simulink model "generator_controls"  (R2021b)
settings: Solver=VariableStepAuto  StartTime=0.0  StopTime=10.0  RelTol=1e-3
libraries: customLib x4, spsAC1AExcitationSystemLib x1, spsDC1AExcitationSystemLib x1, spsST1AExcitationSystemLib x1, eeGovernorG1 x1, eeSmPSS1A x1, eeSmPSS2C x1
settings Model: Creator=JoEn  LastModifiedBy=ah4430
settings DebuggingCC: UnconnectedInputMsg=none  UnconnectedOutputMsg=none  UnconnectedLineMsg=none
settings ModelReferenceCC: EnableRefExpFcnMdlSchedulingChecks=off
settings RTWCC: DLArmComputeVersion=20.02.1

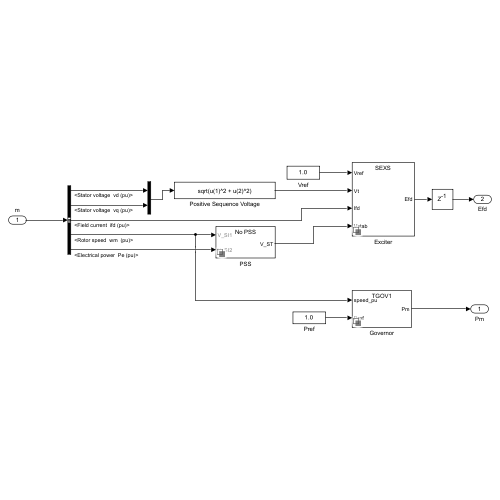
[thumbnail: Simulink's stored preview of the top-level diagram]
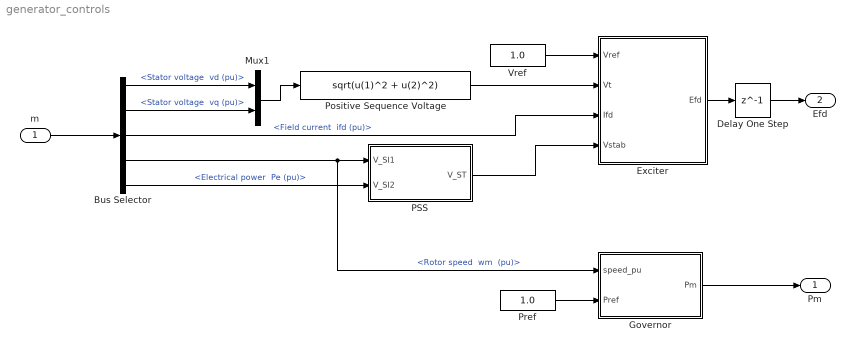
== system generator_controls ==
  m : Inport
  Bus Selector : BusSelector  OutputSignals="dq0 components.Stator voltage  vd (pu),dq0 components.Stator voltage  vq (pu),dq0 components.Field current  ifd (pu),Mechanical.Rotor speed  wm  (pu),Mechanical.Electrical power  Pe (pu)"
  Delay One Step : Delay  DelayLength=1
  Exciter : Subsystem  Variant=on  VariantControlMode=label  LabelModeActiveChoice=sexs
  Governor : Subsystem  Variant=on  VariantControlMode=label  LabelModeActiveChoice=tgov1
  Mux1 : Mux  Inputs=2
  PSS : Subsystem  Variant=on  VariantControlMode=label  LabelModeActiveChoice=none
  Positive Sequence Voltage : Fcn  Expr=sqrt(u(1)^2 + u(2)^2)
  Pref : Constant  Value=1.0
  Vref : Constant  Value=1.0
  Pm : Outport
  Efd : Outport  Port=2
  wires:
  Bus Selector/2 -> Mux1/2  "<Stator voltage  vq (pu)>"
  Vref/1 -> Exciter/1(Vref)
  Delay One Step/1 -> Efd/1
  Bus Selector/3 -> Exciter/3(Ifd)  "<Field current  ifd (pu)>"
  PSS/1(V_ST) -> Exciter/4(Vstab)
  Mux1/1 -> Positive Sequence Voltage/1
  Exciter/1(Efd) -> Delay One Step/1
  Pref/1 -> Governor/2(Pref)
  Governor/1(Pm) -> Pm/1
  Positive Sequence Voltage/1 -> Exciter/2(Vt)
  Bus Selector/1 -> Mux1/1  "<Stator voltage  vd (pu)>"
  m/1 -> Bus Selector/1
  Bus Selector/4 -> Governor/1(speed_pu), PSS/1(V_SI1)  "<Rotor speed  wm  (pu)>"
  Bus Selector/5 -> PSS/2(V_SI2)  "<Electrical power  Pe (pu)>"

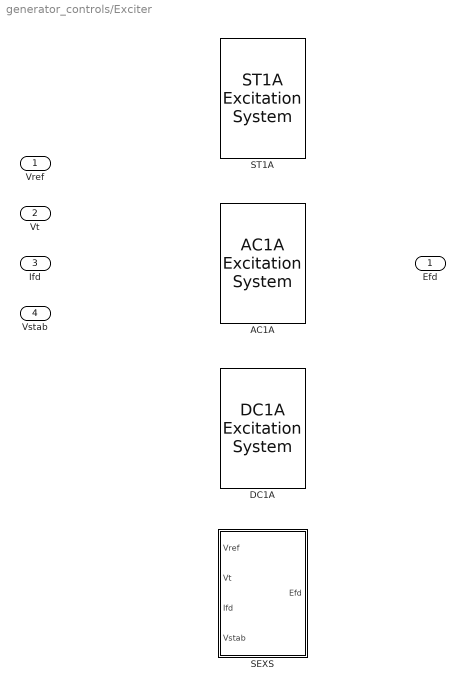
== system generator_controls/Exciter ==
  Vref : Inport
  Vt : Inport  Port=2
  Ifd : Inport  Port=3
  Vstab : Inport  Port=4
  AC1A : spsAC1AExcitationSystemLib/AC1A Excitation System  VariantControl=ac1a  Tr=20e-3  KaTa=[400 0.02]  VAminmax=[-14.5 14.5]  VRminmax=[-5.43 6.03]  KfTf=[0.03 1.0]  TbTc=[0 0]  KeTe=[1.0 0.80]  Ve12=[4.18 3.14]  SeVe12=[0.10 0.03]  Kd=0.38  Kc=0.20  v0=[1.025 1.5083]  TsBlock=0
  DC1A : spsDC1AExcitationSystemLib/DC1A Excitation System  VariantControl=dc1a  Tr=1e-6  KaTa=[20 0.2]  VRminmax=[-5 5]  KfTf=[0.063 0.35]  TbTc=[0 0]  KeTe=[1.0 0.314]  Efd12=[4.5 3.3]  SeEfd12=[4.2662 0.6602]  v0=[1.025 1.5083]  TsBlock=0
  SEXS : Subsystem  VariantControl=sexs
  ST1A : spsST1AExcitationSystemLib/ST1A Excitation System  VariantControl=st1a  Tr=20e-3  KaTa=[210 0.001]  VIminmax=[-999 +999]  VAminmax=[-999 999]  VRminmax=[-6.0 6.43]  KfTf=[0.001 1]  TbTc=[0 0 0 0]  KLR=1  ILR=2  Kc=0.038  v0=[1 1]  TsBlock=0
  Efd : Outport

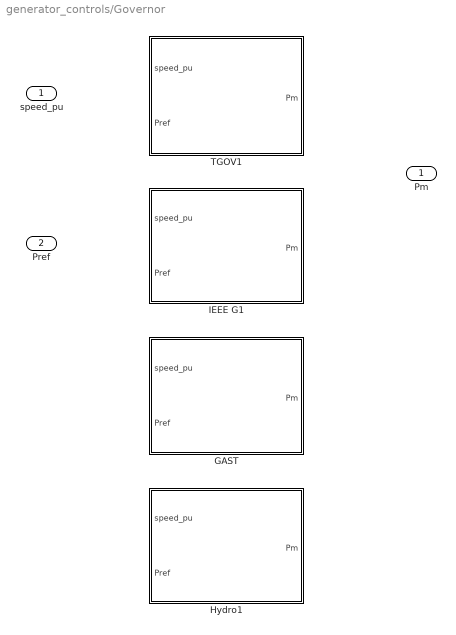
== system generator_controls/Governor ==
  speed_pu : Inport
  Pref : Inport  Port=2
  GAST : Subsystem  VariantControl=gast
  Hydro1 : Subsystem  VariantControl=hydro1
  IEEE G1 : Subsystem  VariantControl=ieeeg1
  TGOV1 : Subsystem  VariantControl=tgov1
  Pm : Outport

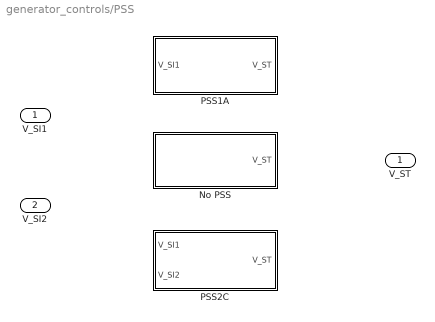
== system generator_controls/PSS ==
  V_SI1 : Inport
  V_SI2 : Inport  Port=2
  No PSS : Subsystem  VariantControl=none
  PSS1A : Subsystem  VariantControl=pss1a
  PSS2C : Subsystem  VariantControl=pss2c
  V_ST : Outport

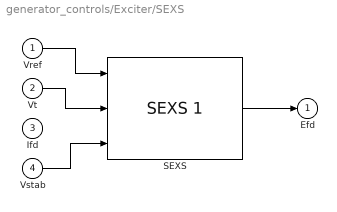
== system generator_controls/Exciter/SEXS ==
  Vref : Inport
  Vt : Inport  Port=2
  Ifd : Inport  Port=3
  Vstab : Inport  Port=4
  SEXS : customLib/SEXS 1  TA=0  TB=0  K=0  TE=0  Emin=0  Emax=0
      settings: SourceProductName=Custom Library
  Efd : Outport
  wires:
  Vref/1 -> SEXS/1
  Vt/1 -> SEXS/2
  Vstab/1 -> SEXS/3
  SEXS/1 -> Efd/1

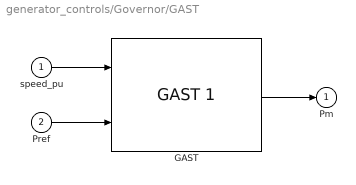
== system generator_controls/Governor/GAST ==
  speed_pu : Inport
  Pref : Inport  Port=2
  GAST : customLib/GAST 1  R=0.05  T_1=0.2  T_2=0.2  T_3=1  A_T=0.5  K_T=1  Vmax=1.1  Vmin=0  DTurb=0
      settings: SourceProductName=Custom Library
  Pm : Outport
  wires:
  Pref/1 -> GAST/2
  speed_pu/1 -> GAST/1
  GAST/1 -> Pm/1

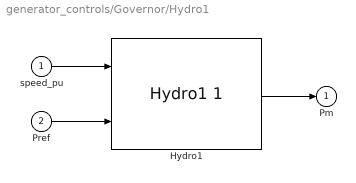
== system generator_controls/Governor/Hydro1 ==
  speed_pu : Inport
  Pref : Inport  Port=2
  Hydro1 : customLib/Hydro1 1  Rt=0.3  TR=5  TF=0.05  TG=0.5  TW=1  AT=10  DT=0.5  QNL=0.08  Rp=0.29  Gmin=0  Gmax=1  Velm=0.2
      settings: SourceProductName=Custom Library
  Pm : Outport
  wires:
  Pref/1 -> Hydro1/2
  speed_pu/1 -> Hydro1/1
  Hydro1/1 -> Pm/1

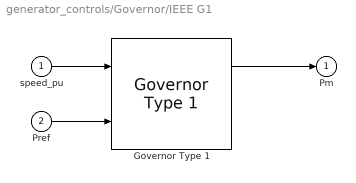
== system generator_controls/Governor/IEEE G1 ==
  speed_pu : Inport
  Pref : Inport  Port=2
  Governor Type 1 : eeGovernorG1/Governor Type 1  pu_speed_reference=1  pu_torque0=0.45  Ts=-1  K=20.4808  T_1=0.78725  T_2=0.57519  T_3=0.31533  U_o=0.10103  U_c=-0.049182  P_max=1.2069  P_min=0.23278  T_4=0.97402  K_1=0.22054  K_2=0  T_5=4.4965  K_3=0.21987  K_4=0  T_6=4.186  K_5=0.30004  K_6=0  T_7=1.7521  K_7=0.25973  K_8=0  db1=0.02
  Pm : Outport
  wires:
  Pref/1 -> Governor Type 1/2
  speed_pu/1 -> Governor Type 1/1
  Governor Type 1/1 -> Pm/1

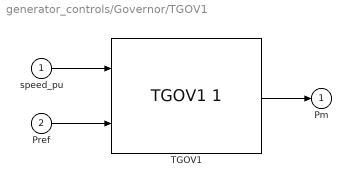
== system generator_controls/Governor/TGOV1 ==
  speed_pu : Inport
  Pref : Inport  Port=2
  TGOV1 : customLib/TGOV1 1  R=0.05  T_1=0.05  Vmax=5  Vmin=-5  T_2=2.1  T_3=7  Dt=0
      settings: SourceProductName=Custom Library
  Pm : Outport
  wires:
  Pref/1 -> TGOV1/2
  speed_pu/1 -> TGOV1/1
  TGOV1/1 -> Pm/1

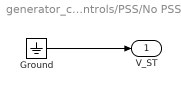
== system generator_controls/PSS/No PSS ==
  Ground : Ground
  V_ST : Outport
  wires:
  Ground/1 -> V_ST/1

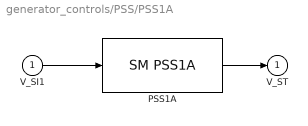
== system generator_controls/PSS/PSS1A ==
  V_SI1 : Inport
  PSS1A : eeSmPSS1A/SM PSS1A  K_S=3.1525  A_1=0.028257  A_2=1.0467  T_1=0.76  T_2=0.087367  T_3=0.76014  T_4=0.023652  T_5=9.8466  T_6=0.021582  V_STmax=0.09037  V_STmin=-0.076348  Ts=-1
  V_ST : Outport
  wires:
  V_SI1/1 -> PSS1A/1
  PSS1A/1 -> V_ST/1

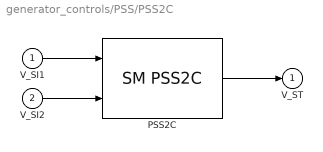
== system generator_controls/PSS/PSS2C ==
  V_SI1 : Inport
  V_SI2 : Inport  Port=2
  PSS2C : eeSmPSS2C/SM PSS2C  K_S1=5  K_S2=1.4184  K_S3=1  T_6=0  T_7=10  T_w1=10  T_w2=10  T_w3=10  T_w4=0  T_8=0.5  T_9=0.1  M=5  N=1  T_1=0.16  T_2=0.04  T_3=0.16  T_4=0.04  T_10=0.18  T_11=0.03  T_12=0  T_13=0  V_STmax=0.1  V_STmin=-0.1  V_SI1max=2  V_SI1min=-2  V_SI2max=2  V_SI2min=-2  P_PSSon=0  P_PSSoff=0  Ts=-1
  V_ST : Outport
  wires:
  V_SI1/1 -> PSS2C/1
  PSS2C/1 -> V_ST/1
  V_SI2/1 -> PSS2C/2
